simulink model "motorCooling"  (R2022b)
settings: Solver=VariableStepAuto  StartTime=0.0  StopTime=80  RelTol=1e-3  AbsTol=1e-3
PreLoadFcn:
  | load fsDCycle.mat
  | vehicleData
undefined symbols (not defined in the file or in its folder): battery, bevGear, bevMotorSpdRef, cooling, FL, FR, motorDrive, RL, RR, vehicle
libraries: fl_lib x47, nesl_utility x24, sdl_lib x11, SimscapeFluids_lib x3, ee_lib x2, simulink x1, slpidlib x1, autolibshared x1, batteryecm_lib x1, BatteryEstimators x1
(part 3 of 3)

== system motorCooling/Vehicle/Electric Powertrain/SOC ==
  Constant1 : Constant  Value=battery.init_soc
  Current Sensor : fl_lib/Electrical/Electrical Sensors/Current Sensor
  Gain : Gain  Gain=-1
  PS-Simulink Converter1 : nesl_utility/PS-Simulink Converter  PhysicalDomain=network_engine_domain  SubClassName=ps_output  LeftPortType=input  RightPortType=output  PseudoPeriodic=off  Frequencies=[]  VectorFormat=1-D array  Unit=A  AffineConversion=off
  SOC Estimator (Coulomb Counting) : BatteryEstimators/SOC Estimator (Coulomb Counting)  AH=20  Ts=-1
      link override Integrator: LabelModeActiveChoice=Discrete
      settings: LibrarySourceBlock=|
      | batt_sl_lib/Estimators/SOC Estimator
      | (Coulomb Counting)
  + : PMIOPort  Side=Left
  - : PMIOPort  Port=2  Side=Right
  tag scope: SOC=global
  wires:
  Constant1/1 -> SOC Estimator (Coulomb Counting)/2
  SOC Estimator (Coulomb Counting)/1 -> [SOC]  "SOC"
  Gain/1 -> SOC Estimator (Coulomb Counting)/1
  PS-Simulink Converter1/1 -> Gain/1
  connections:
  Current Sensor/RConn2 -- -/RConn1
  PS-Simulink Converter1/LConn1 -- Current Sensor/RConn1
  Current Sensor/LConn1 -- +/RConn1

== system motorCooling/Vehicle/Electric Powertrain/Speed Sensor ==
  Mechanical Rotational Reference1 : fl_lib/Mechanical/Rotational Elements/Mechanical Rotational Reference
  Motion Sensor : fl_lib/Mechanical/Mechanical Sensors/Ideal Rotational Motion Sensor  reference=foundation.enum.MeasurementReference.difference  acceleration_port=false  velocity_port=true  position_port=true  wrap_angle=simscape.enum.onoff.off  offset=0 rad
  PS Terminator : fl_lib/Physical Signals/Sinks/PS Terminator
  PS-Simulink Converter 2 : nesl_utility/PS-Simulink Converter  PhysicalDomain=network_engine_domain  SubClassName=ps_output  LeftPortType=input  RightPortType=output  PseudoPeriodic=off  Frequencies=[]  VectorFormat=1-D array  Unit=rpm  AffineConversion=off
  R : PMIOPort  Side=Left
  w : Outport
  wires:
  PS-Simulink Converter 2/1 -> w/1
  connections:
  Motion Sensor/RConn2 -- PS-Simulink Converter 2/LConn1
  Motion Sensor/RConn1 -- Mechanical Rotational Reference1/LConn1
  Motion Sensor/RConn3 -- PS Terminator/LConn1
  Motion Sensor/LConn1 -- R/RConn1

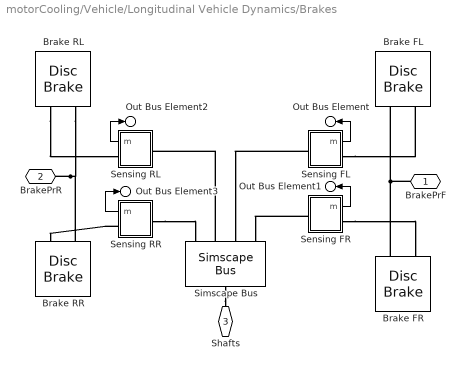
== system motorCooling/Vehicle/Longitudinal Vehicle Dynamics/Brakes ==
  Brake FL : sdl_lib/Brakes & Detents/Rotational/Disc Brake  r_mean=brake.padRadius mm  bore=brake.cylinderBore mm  n_pads=1  thermal_port=simscape.enum.thermaleffects.omit  mu_static=brake.sf  mu_coulomb=brake.cf  temperature_TLU=[280, 300, 320] K  mu_static_TLU=[.9, .8, .7]  mu_coulomb_TLU=[.8, .7, .6]  brkwy_vel=brake.frictionVel rad/s  visc_coef=brake.vfc N*m*s/rad  enable_faults=simscape.enum.onoff.off  faulted_pressure=0 bar  external_fault=simscape.enum.onoff.off  temporal_fault=simscape.enum.onoff.off  fault_time=5 s  report_fault=simscape.enum.assert.action.none  thermal_mass=50 kJ/K  temperature_specify=off  temperature_priority=High  temperature=300 K  temperature_nominal_specify=off  temperature_nominal_unit=K  temperature_nominal_value=1
  Brake FR : sdl_lib/Brakes & Detents/Rotational/Disc Brake  r_mean=brake.padRadius mm  bore=brake.cylinderBore mm  n_pads=1  thermal_port=simscape.enum.thermaleffects.omit  mu_static=brake.sf  mu_coulomb=brake.cf  temperature_TLU=[280, 300, 320] K  mu_static_TLU=[.9, .8, .7]  mu_coulomb_TLU=[.8, .7, .6]  brkwy_vel=brake.frictionVel rad/s  visc_coef=brake.vfc N*m*s/rad  enable_faults=simscape.enum.onoff.off  faulted_pressure=0 bar  external_fault=simscape.enum.onoff.off  temporal_fault=simscape.enum.onoff.off  fault_time=5 s  report_fault=simscape.enum.assert.action.none  thermal_mass=50 kJ/K  temperature_specify=off  temperature_priority=High  temperature=300 K  temperature_nominal_specify=off  temperature_nominal_unit=K  temperature_nominal_value=1
  Brake RL : sdl_lib/Brakes & Detents/Rotational/Disc Brake  r_mean=brake.padRadius mm  bore=brake.cylinderBore mm  n_pads=1  thermal_port=simscape.enum.thermaleffects.omit  mu_static=brake.sf  mu_coulomb=brake.cf  temperature_TLU=[280, 300, 320] K  mu_static_TLU=[.9, .8, .7]  mu_coulomb_TLU=[.8, .7, .6]  brkwy_vel=brake.frictionVel rad/s  visc_coef=brake.vfc N*m*s/rad  enable_faults=simscape.enum.onoff.off  faulted_pressure=0 bar  external_fault=simscape.enum.onoff.off  temporal_fault=simscape.enum.onoff.off  fault_time=5 s  report_fault=simscape.enum.assert.action.none  thermal_mass=50 kJ/K  temperature_specify=off  temperature_priority=High  temperature=300 K  temperature_nominal_specify=off  temperature_nominal_unit=K  temperature_nominal_value=1
  Brake RR : sdl_lib/Brakes & Detents/Rotational/Disc Brake  r_mean=brake.padRadius mm  bore=brake.cylinderBore mm  n_pads=1  thermal_port=simscape.enum.thermaleffects.omit  mu_static=brake.sf  mu_coulomb=brake.cf  temperature_TLU=[280, 300, 320] K  mu_static_TLU=[.9, .8, .7]  mu_coulomb_TLU=[.8, .7, .6]  brkwy_vel=brake.frictionVel rad/s  visc_coef=brake.vfc N*m*s/rad  enable_faults=simscape.enum.onoff.off  faulted_pressure=0 bar  external_fault=simscape.enum.onoff.off  temporal_fault=simscape.enum.onoff.off  fault_time=5 s  report_fault=simscape.enum.assert.action.none  thermal_mass=50 kJ/K  temperature_specify=off  temperature_priority=High  temperature=300 K  temperature_nominal_specify=off  temperature_nominal_unit=K  temperature_nominal_value=1
  Sensing FL : Subsystem
  Sensing FR : Subsystem
  Sensing RL : Subsystem
  Sensing RR : Subsystem
  Simscape Bus : SimscapeBus  HierarchyStrings=RR;RL;FL;FR
  BrakePrF : PMIOPort  Side=Left
  BrakePrR : PMIOPort  Port=2  Side=Left
  Shafts : PMIOPort  Port=3  Side=Right
  Out Bus Element : Outport  PortName=m  Element=FL
  Out Bus Element1 : Outport  PortName=m  Element=FR
  Out Bus Element2 : Outport  PortName=m  Element=RL
  Out Bus Element3 : Outport  PortName=m  Element=RR
  wires:
  Sensing FL/1(m) -> Out Bus Element/1
  Sensing FR/1(m) -> Out Bus Element1/1
  Sensing RL/1(m) -> Out Bus Element2/1
  Sensing RR/1(m) -> Out Bus Element3/1
  connections:
  BrakePrR/RConn1 -- Brake RL/LConn1 -- Brake RR/LConn1
  Brake FR/LConn1 -- Brake FL/LConn1 -- BrakePrF/RConn1
  Sensing FL/LConn1 -- Simscape Bus/LConn3
  Sensing FR/LConn1 -- Simscape Bus/LConn4
  Simscape Bus/LConn2 -- Sensing RL/LConn1
  Sensing RR/LConn1 -- Simscape Bus/LConn1
  Simscape Bus/RConn1 -- Shafts/RConn1
  Sensing FL/RConn1 -- Brake FL/LConn2
  Sensing FR/RConn1 -- Brake FR/LConn2
  Brake RL/LConn2 -- Sensing RL/RConn1
  Sensing RR/RConn1 -- Brake RR/LConn2

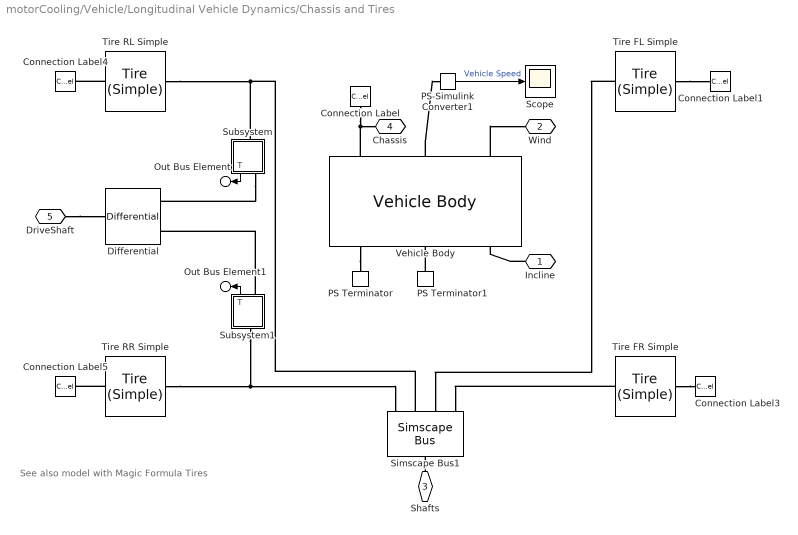
== system motorCooling/Vehicle/Longitudinal Vehicle Dynamics/Chassis and Tires ==
  note: See also model with Magic Formula Tires
  Connection Label{,1,3..5} (5 alike) : ConnectionLabel  Label=VehicleHub
  Differential : sdl_lib/Gears/Differential  driveshaft_location=sdl.enum.differential_orientation.right  cd_ratio=bevGear.gearRatio  friction_model=sdl.enum.gear_friction.none  efficiency=[.85, .92]  temperature_TLU=[280, 300, 320] K  efficiency_ss_TLU=[.95, .9, .85]  efficiency_cd_TLU=[.95, .9, .85]  pwr_thr=[.001, .001] W  mu_visc=[0, 0] N*m*s/rad  model_inertia=simscape.enum.onoff.off  carrier_inertia=0.001 kg*m^2  planet_inertia=0.001 kg*m^2  thermal_mass=50 J/K  T_init=300 K
  PS Terminator : fl_lib/Physical Signals/Sinks/PS Terminator
  PS Terminator1 : fl_lib/Physical Signals/Sinks/PS Terminator
  PS-Simulink Converter1 : nesl_utility/PS-Simulink Converter  PhysicalDomain=network_engine_domain  SubClassName=ps_output  LeftPortType=input  RightPortType=output  PseudoPeriodic=off  Frequencies=[]  VectorFormat=1-D array  Unit=1  AffineConversion=off
  Scope : Scope
  Simscape Bus1 : SimscapeBus  HierarchyStrings=RR;RL;FL;FR
  Subsystem : Subsystem
  Subsystem1 : Subsystem
  Tire FL Simple : sdl_lib/Tires & Vehicles/Tire (Simple)  r_tire=vehicle.tireRollingRadius_cm cm  model_compliance=sdl.enum.compliance.off  stiffness=1e6 N/m  damping=1000 N*s/m  model_inertia=sdl.enum.model_inertia.off  tire_inertia=1 kg*m^2  initial_velocity=0 rad/s
      settings: InternalSimscapePortConfiguration="{\"Bottom\":[],\"Left\":[{\"id\":\"A\",\"label\":\"A\",\"type\":\"foundation.mechanical.rotational.rotational\"}],\"Right\":[{\"id\":\"H\",\"label\":\"H\",\"type\":\"foundation.mechanical.translational.translational\"}],\"Top\":[]}"
  Tire FR Simple : sdl_lib/Tires & Vehicles/Tire (Simple)  r_tire=vehicle.tireRollingRadius_cm cm  model_compliance=sdl.enum.compliance.off  stiffness=1e6 N/m  damping=1000 N*s/m  model_inertia=sdl.enum.model_inertia.off  tire_inertia=1 kg*m^2  initial_velocity=0 rad/s
      settings: InternalSimscapePortConfiguration="{\"Bottom\":[],\"Left\":[{\"id\":\"A\",\"label\":\"A\",\"type\":\"foundation.mechanical.rotational.rotational\"}],\"Right\":[{\"id\":\"H\",\"label\":\"H\",\"type\":\"foundation.mechanical.translational.translational\"}],\"Top\":[]}"
  Tire RL Simple : sdl_lib/Tires & Vehicles/Tire (Simple)  r_tire=vehicle.tireRollingRadius_cm cm  model_compliance=sdl.enum.compliance.off  stiffness=1e6 N/m  damping=1000 N*s/m  model_inertia=sdl.enum.model_inertia.off  tire_inertia=1 kg*m^2  initial_velocity=0 rad/s
      settings: InternalSimscapePortConfiguration="{\"Bottom\":[],\"Left\":[{\"id\":\"A\",\"label\":\"A\",\"type\":\"foundation.mechanical.rotational.rotational\"}],\"Right\":[{\"id\":\"H\",\"label\":\"H\",\"type\":\"foundation.mechanical.translational.translational\"}],\"Top\":[]}"
  Tire RR Simple : sdl_lib/Tires & Vehicles/Tire (Simple)  r_tire=vehicle.tireRollingRadius_cm cm  model_compliance=sdl.enum.compliance.off  stiffness=1e6 N/m  damping=1000 N*s/m  model_inertia=sdl.enum.model_inertia.off  tire_inertia=1 kg*m^2  initial_velocity=0 rad/s
      settings: InternalSimscapePortConfiguration="{\"Bottom\":[],\"Left\":[{\"id\":\"A\",\"label\":\"A\",\"type\":\"foundation.mechanical.rotational.rotational\"}],\"Right\":[{\"id\":\"H\",\"label\":\"H\",\"type\":\"foundation.mechanical.translational.translational\"}],\"Top\":[]}"
  Vehicle Body : sdl_lib/Tires & Vehicles/Vehicle Body  mass=vehicle.riderMass + vehicle.vehicleMass kg  n_w=2  x_f=vehicle.frontAxleDis mm  x_r=vehicle.rearAxleDis mm  y_c=vehicle.cgHeight mm  mass_var=simscape.enum.onoff.off  g=9.81 m/s^2  liftoff_warning=simscape.enum.onoff.off  area=vehicle.frontalArea m^2  Cd=vehicle.cd  rho=1.18 kg/m^3  model_pitch=simscape.enum.onoff.off  inertia=4000 kg*m^2  suspension_model=sdl.enum.linearTLU.linear  k_f=1e4 N/m  b_f=1e4 N*s/m  k_r=1e4 N/m  b_r=1e4 N*s/m  k_f_TLU=[-2000, -1000, 0, 1000, 2000] N  x_f_TLU=[-.4, -.2, 0, .2, .4] m  b_f_TLU=[-200, -100, 0, 100, 200] N  v_f_TLU=[-4, -2, 0, 2, 4] m/s  k_r_TLU=[-2000, -1000, 0, 1000, 2000] N  x_r_TLU=[-.4, -.2, 0, .2, .4] m  b_r_TLU=[-200, -100, 0, 100, 200] N  v_r_TLU=[-4, -2, 0, 2, 4] m/s  interp_method=simscape.enum.interpolation.linear  extrap_method=simscape.enum.extrapolation.linear  model_hardstop=simscape.enum.onoff.off  upper_bound_f=.25 m  lower_bound_f=-.25 m  stop_k_f=1e6 N/m  stop_b_f=150 N*s/m  upper_bound_r=.25 m  lower_bound_r=-.25 m  stop_k_r=1e6 N/m  stop_b_r=150 N*s/m  initial_pitch=0 rad  initial_pitch_rate=0 rad/s  v_specify=off  v_priority=High  v=12.95 m/s  v_nominal_specify=off  v_nominal_unit=m/s  v_nominal_value=1
  Incline : PMIOPort  Side=Right
  Wind : PMIOPort  Port=2  Side=Right
  Shafts : PMIOPort  Port=3  Side=Left
  Chassis : PMIOPort  Port=4  Side=Right
  DriveShaft : PMIOPort  Port=5  Side=Left
  Out Bus Element : Outport  PortName=m  Element=tRL
  Out Bus Element1 : Outport  PortName=m  Element=tRR
  wires:
  PS-Simulink Converter1/1 -> Scope/1  "Vehicle Speed"
  Subsystem/1(T) -> Out Bus Element/1
  Subsystem1/1(T) -> Out Bus Element1/1
  connections:
  Tire RR Simple/RConn1 -- Connection Label5/LConn1
  Tire FL Simple/RConn1 -- Connection Label1/LConn1
  Tire RL Simple/RConn1 -- Connection Label4/LConn1
  Vehicle Body/LConn2 -- PS-Simulink Converter1/LConn1
  Tire FR Simple/RConn1 -- Connection Label3/LConn1
  Tire FR Simple/LConn1 -- Simscape Bus1/LConn4
  DriveShaft/RConn1 -- Differential/LConn1
  Connection Label/LConn1 -- Vehicle Body/LConn1 -- Chassis/RConn1
  Subsystem1/LConn1 -- Tire RR Simple/LConn1 -- Simscape Bus1/LConn1
  Tire FL Simple/LConn1 -- Simscape Bus1/LConn3
  Simscape Bus1/LConn2 -- Tire RL Simple/LConn1 -- Subsystem/LConn1
  Shafts/RConn1 -- Simscape Bus1/RConn1
  Incline/RConn1 -- Vehicle Body/RConn3
  Vehicle Body/LConn3 -- Wind/RConn1
  Subsystem1/RConn1 -- Differential/RConn1
  Subsystem/RConn1 -- Differential/RConn2
  Vehicle Body/RConn1 -- PS Terminator/LConn1
  PS Terminator1/LConn1 -- Vehicle Body/RConn2

== system motorCooling/Vehicle/Longitudinal Vehicle Dynamics/Env ==
  m : Inport
  Road Grade (rad) : Constant  Value=0
  Signal Specification : SignalSpecification  Unit=rad
  Terminator : Terminator
  Wind (m/s) : Constant  Value=0
  Bus Element Out2 : Outport  PortName=Env  Element=RoadGrade
      settings: AttributesFormatString=%<Unit>
  Bus Element Out4 : Outport  PortName=Env  Element=Wind
      settings: AttributesFormatString=%<Unit>
  wires:
  Wind (m/s)/1 -> Bus Element Out4/1
  m/1 -> Terminator/1
  Road Grade (rad)/1 -> Signal Specification/1
  Signal Specification/1 -> Bus Element Out2/1

== system motorCooling/Vehicle/Longitudinal Vehicle Dynamics/Pressure Drag ==
  Vel : Inport
  Gain : Gain  Gain=0.5*cooling.cDrag*cooling.denAir
  Simulink-PS Converter : nesl_utility/Simulink-PS Converter  PhysicalDomain=network_engine_domain  SubClassName=ps_input  LeftPortType=input  RightPortType=output  PseudoPeriodic=off  Frequencies=[]  NoiseDistribution=none  NoiseParameters=[]  Unit=Pa  AffineConversion=off  FilteringAndDerivatives=provide  SimscapeFilterOrder=1  InputFilterTimeConstant=0.001  UdotUserProvided=0
  Square : Math  Operator=square
  Transfer Fcn : TransferFcn  Denominator=[0.5 1]
  Pressure : PMIOPort  Side=Right
  wires:
  Vel/1 -> Square/1
  Gain/1 -> Transfer Fcn/1
  Square/1 -> Gain/1
  Transfer Fcn/1 -> Simulink-PS Converter/1
  connections:
  Simulink-PS Converter/RConn1 -- Pressure/RConn1

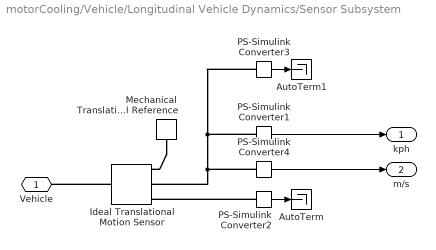
== system motorCooling/Vehicle/Longitudinal Vehicle Dynamics/Sensor Subsystem ==
  AutoTerm : Terminator
  AutoTerm1 : Terminator
  Ideal Translational Motion Sensor : fl_lib/Mechanical/Mechanical Sensors/Ideal Translational Motion Sensor  reference=foundation.enum.MeasurementReference.difference  acceleration_port=false  velocity_port=true  position_port=true  offset=0 m
  Mechanical Translational Reference : fl_lib/Mechanical/Translational Elements/Mechanical Translational Reference
  PS-Simulink Converter1 : nesl_utility/PS-Simulink Converter  PhysicalDomain=network_engine_domain  SubClassName=ps_output  LeftPortType=input  RightPortType=output  PseudoPeriodic=off  Frequencies=[]  VectorFormat=1-D array  Unit=km/hr  AffineConversion=off
  PS-Simulink Converter2 : nesl_utility/PS-Simulink Converter  PhysicalDomain=network_engine_domain  SubClassName=ps_output  LeftPortType=input  RightPortType=output  PseudoPeriodic=off  Frequencies=[]  VectorFormat=1-D array  Unit=1  AffineConversion=off
  PS-Simulink Converter3 : nesl_utility/PS-Simulink Converter  PhysicalDomain=network_engine_domain  SubClassName=ps_output  LeftPortType=input  RightPortType=output  PseudoPeriodic=off  Frequencies=[]  VectorFormat=1-D array  Unit=mph  AffineConversion=off
  PS-Simulink Converter4 : nesl_utility/PS-Simulink Converter  PhysicalDomain=network_engine_domain  SubClassName=ps_output  LeftPortType=input  RightPortType=output  PseudoPeriodic=off  Frequencies=[]  VectorFormat=1-D array  Unit=m/s  AffineConversion=off
  Vehicle : PMIOPort  Side=Left
  kph : Outport  VectorParamsAs1DForOutWhenUnconnected=off
  m/s : Outport  Port=2  VectorParamsAs1DForOutWhenUnconnected=off
  wires:
  PS-Simulink Converter1/1 -> kph/1
  PS-Simulink Converter2/1 -> AutoTerm/1
  PS-Simulink Converter3/1 -> AutoTerm1/1
  PS-Simulink Converter4/1 -> m/s/1
  connections:
  Mechanical Translational Reference/LConn1 -- Ideal Translational Motion Sensor/RConn1
  PS-Simulink Converter2/LConn1 -- Ideal Translational Motion Sensor/RConn3
  Ideal Translational Motion Sensor/LConn1 -- Vehicle/RConn1
  PS-Simulink Converter3/LConn1 -- PS-Simulink Converter4/LConn1 -- Ideal Translational Motion Sensor/RConn2 -- PS-Simulink Converter1/LConn1

== system motorCooling/Vehicle/Electric Powertrain/Motor Cooling System/Sensing Temperature ==
  PS-Simulink Converter : nesl_utility/PS-Simulink Converter  PhysicalDomain=network_engine_domain  SubClassName=ps_output  LeftPortType=input  RightPortType=output  PseudoPeriodic=off  Frequencies=[]  VectorFormat=inherit  Unit=degC  AffineConversion=on
  Temperature Sensor : fl_lib/Thermal/Thermal Sensors/Temperature Sensor
  Thermal Reference : fl_lib/Thermal/Thermal Elements/Thermal Reference
  H : PMIOPort  Side=Left
  T : Outport
  wires:
  PS-Simulink Converter/1 -> T/1  "Motor Temperature"
  connections:
  PS-Simulink Converter/LConn1 -- Temperature Sensor/RConn2
  Thermal Reference/LConn1 -- Temperature Sensor/RConn1
  Temperature Sensor/LConn1 -- H/RConn1

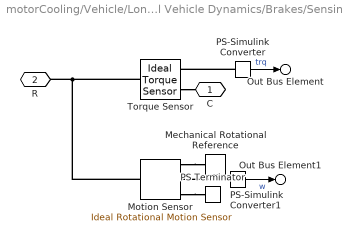
== system motorCooling/Vehicle/Longitudinal Vehicle Dynamics/Brakes/Sensing FL ==
  Mechanical Rotational Reference : fl_lib/Mechanical/Rotational Elements/Mechanical Rotational Reference
  Motion Sensor : fl_lib/Mechanical/Mechanical Sensors/Ideal Rotational Motion Sensor  reference=foundation.enum.MeasurementReference.difference  acceleration_port=false  velocity_port=true  position_port=true  wrap_angle=simscape.enum.onoff.off  offset=0 rad
  PS Terminator : fl_lib/Physical Signals/Sinks/PS Terminator
  PS-Simulink Converter : nesl_utility/PS-Simulink Converter  PhysicalDomain=network_engine_domain  SubClassName=ps_output  LeftPortType=input  RightPortType=output  PseudoPeriodic=off  Frequencies=[]  VectorFormat=inherit  Unit=inherit  AffineConversion=off
  PS-Simulink Converter1 : nesl_utility/PS-Simulink Converter  PhysicalDomain=network_engine_domain  SubClassName=ps_output  LeftPortType=input  RightPortType=output  PseudoPeriodic=off  Frequencies=[]  VectorFormat=inherit  Unit=inherit  AffineConversion=off
  Torque Sensor : fl_lib/Mechanical/Mechanical Sensors/Ideal Torque Sensor
  C : PMIOPort  Side=Left
  R : PMIOPort  Port=2  Side=Right
  Out Bus Element : Outport  PortName=m  Element=brkTrqFL
  Out Bus Element1 : Outport  PortName=m  Element=wFL
  wires:
  PS-Simulink Converter1/1 -> Out Bus Element1/1  "w"
  PS-Simulink Converter/1 -> Out Bus Element/1  "trq"
  connections:
  Motion Sensor/RConn3 -- PS Terminator/LConn1
  PS-Simulink Converter1/LConn1 -- Motion Sensor/RConn2
  Motion Sensor/RConn1 -- Mechanical Rotational Reference/LConn1
  Torque Sensor/RConn1 -- C/RConn1
  Motion Sensor/LConn1 -- Torque Sensor/LConn1 -- R/RConn1
  PS-Simulink Converter/LConn1 -- Torque Sensor/RConn2

== system motorCooling/Vehicle/Longitudinal Vehicle Dynamics/Brakes/Sensing FR ==
  Mechanical Rotational Reference : fl_lib/Mechanical/Rotational Elements/Mechanical Rotational Reference
  Motion Sensor : fl_lib/Mechanical/Mechanical Sensors/Ideal Rotational Motion Sensor  reference=foundation.enum.MeasurementReference.difference  acceleration_port=false  velocity_port=true  position_port=true  wrap_angle=simscape.enum.onoff.off  offset=0 rad
  PS Terminator : fl_lib/Physical Signals/Sinks/PS Terminator
  PS-Simulink Converter : nesl_utility/PS-Simulink Converter  PhysicalDomain=network_engine_domain  SubClassName=ps_output  LeftPortType=input  RightPortType=output  PseudoPeriodic=off  Frequencies=[]  VectorFormat=inherit  Unit=inherit  AffineConversion=off
  PS-Simulink Converter1 : nesl_utility/PS-Simulink Converter  PhysicalDomain=network_engine_domain  SubClassName=ps_output  LeftPortType=input  RightPortType=output  PseudoPeriodic=off  Frequencies=[]  VectorFormat=inherit  Unit=inherit  AffineConversion=off
  Torque Sensor : fl_lib/Mechanical/Mechanical Sensors/Ideal Torque Sensor
  C : PMIOPort  Side=Left
  R : PMIOPort  Port=2  Side=Right
  Out Bus Element : Outport  PortName=m  Element=brkTrqFR
  Out Bus Element1 : Outport  PortName=m  Element=wFR
  wires:
  PS-Simulink Converter/1 -> Out Bus Element/1  "trq"
  PS-Simulink Converter1/1 -> Out Bus Element1/1  "w"
  connections:
  PS-Simulink Converter/LConn1 -- Torque Sensor/RConn2
  R/RConn1 -- Torque Sensor/LConn1 -- Motion Sensor/LConn1
  Torque Sensor/RConn1 -- C/RConn1
  Motion Sensor/RConn1 -- Mechanical Rotational Reference/LConn1
  PS-Simulink Converter1/LConn1 -- Motion Sensor/RConn2
  Motion Sensor/RConn3 -- PS Terminator/LConn1

== system motorCooling/Vehicle/Longitudinal Vehicle Dynamics/Brakes/Sensing RL ==
  Mechanical Rotational Reference : fl_lib/Mechanical/Rotational Elements/Mechanical Rotational Reference
  Motion Sensor : fl_lib/Mechanical/Mechanical Sensors/Ideal Rotational Motion Sensor  reference=foundation.enum.MeasurementReference.difference  acceleration_port=false  velocity_port=true  position_port=true  wrap_angle=simscape.enum.onoff.off  offset=0 rad
  PS Terminator : fl_lib/Physical Signals/Sinks/PS Terminator
  PS-Simulink Converter : nesl_utility/PS-Simulink Converter  PhysicalDomain=network_engine_domain  SubClassName=ps_output  LeftPortType=input  RightPortType=output  PseudoPeriodic=off  Frequencies=[]  VectorFormat=inherit  Unit=inherit  AffineConversion=off
  PS-Simulink Converter1 : nesl_utility/PS-Simulink Converter  PhysicalDomain=network_engine_domain  SubClassName=ps_output  LeftPortType=input  RightPortType=output  PseudoPeriodic=off  Frequencies=[]  VectorFormat=inherit  Unit=inherit  AffineConversion=off
  Torque Sensor : fl_lib/Mechanical/Mechanical Sensors/Ideal Torque Sensor
  C : PMIOPort  Side=Left
  R : PMIOPort  Port=2  Side=Right
  Out Bus Element : Outport  PortName=m  Element=brkTrqRL
  Out Bus Element1 : Outport  PortName=m  Element=wRL
  wires:
  PS-Simulink Converter/1 -> Out Bus Element/1  "trq"
  PS-Simulink Converter1/1 -> Out Bus Element1/1  "w"
  connections:
  PS-Simulink Converter/LConn1 -- Torque Sensor/RConn2
  Torque Sensor/LConn1 -- Motion Sensor/LConn1 -- R/RConn1
  Torque Sensor/RConn1 -- C/RConn1
  Motion Sensor/RConn1 -- Mechanical Rotational Reference/LConn1
  PS-Simulink Converter1/LConn1 -- Motion Sensor/RConn2
  Motion Sensor/RConn3 -- PS Terminator/LConn1

== system motorCooling/Vehicle/Longitudinal Vehicle Dynamics/Brakes/Sensing RR ==
  Mechanical Rotational Reference : fl_lib/Mechanical/Rotational Elements/Mechanical Rotational Reference
  Motion Sensor : fl_lib/Mechanical/Mechanical Sensors/Ideal Rotational Motion Sensor  reference=foundation.enum.MeasurementReference.difference  acceleration_port=false  velocity_port=true  position_port=true  wrap_angle=simscape.enum.onoff.off  offset=0 rad
  PS Terminator : fl_lib/Physical Signals/Sinks/PS Terminator
  PS-Simulink Converter : nesl_utility/PS-Simulink Converter  PhysicalDomain=network_engine_domain  SubClassName=ps_output  LeftPortType=input  RightPortType=output  PseudoPeriodic=off  Frequencies=[]  VectorFormat=inherit  Unit=inherit  AffineConversion=off
  PS-Simulink Converter1 : nesl_utility/PS-Simulink Converter  PhysicalDomain=network_engine_domain  SubClassName=ps_output  LeftPortType=input  RightPortType=output  PseudoPeriodic=off  Frequencies=[]  VectorFormat=inherit  Unit=inherit  AffineConversion=off
  Torque Sensor : fl_lib/Mechanical/Mechanical Sensors/Ideal Torque Sensor
  C : PMIOPort  Side=Left
  R : PMIOPort  Port=2  Side=Right
  Out Bus Element : Outport  PortName=m  Element=brqTrqRR
  Out Bus Element1 : Outport  PortName=m  Element=wRR
  wires:
  PS-Simulink Converter1/1 -> Out Bus Element1/1  "w"
  PS-Simulink Converter/1 -> Out Bus Element/1  "trq"
  connections:
  Motion Sensor/RConn3 -- PS Terminator/LConn1
  PS-Simulink Converter1/LConn1 -- Motion Sensor/RConn2
  Motion Sensor/RConn1 -- Mechanical Rotational Reference/LConn1
  Torque Sensor/RConn1 -- C/RConn1
  Motion Sensor/LConn1 -- Torque Sensor/LConn1 -- R/RConn1
  PS-Simulink Converter/LConn1 -- Torque Sensor/RConn2

== system motorCooling/Vehicle/Longitudinal Vehicle Dynamics/Chassis and Tires/Subsystem ==
  PS-Simulink Converter : nesl_utility/PS-Simulink Converter  PhysicalDomain=network_engine_domain  SubClassName=ps_output  LeftPortType=input  RightPortType=output  PseudoPeriodic=off  Frequencies=[]  VectorFormat=inherit  Unit=inherit  AffineConversion=off
  Torque Sensor Motor RL : fl_lib/Mechanical/Mechanical Sensors/Ideal Torque Sensor
  C : PMIOPort  Side=Left
  R : PMIOPort  Port=2  Side=Right
  T : Outport
  wires:
  PS-Simulink Converter/1 -> T/1
  connections:
  Torque Sensor Motor RL/RConn1 -- C/RConn1
  Torque Sensor Motor RL/LConn1 -- R/RConn1
  PS-Simulink Converter/LConn1 -- Torque Sensor Motor RL/RConn2

== system motorCooling/Vehicle/Longitudinal Vehicle Dynamics/Chassis and Tires/Subsystem1 ==
  PS-Simulink Converter : nesl_utility/PS-Simulink Converter  PhysicalDomain=network_engine_domain  SubClassName=ps_output  LeftPortType=input  RightPortType=output  PseudoPeriodic=off  Frequencies=[]  VectorFormat=inherit  Unit=inherit  AffineConversion=off
  Torque Sensor Motor RL : fl_lib/Mechanical/Mechanical Sensors/Ideal Torque Sensor
  C : PMIOPort  Side=Left
  R : PMIOPort  Port=2  Side=Right
  T : Outport
  wires:
  PS-Simulink Converter/1 -> T/1
  connections:
  PS-Simulink Converter/LConn1 -- Torque Sensor Motor RL/RConn2
  Torque Sensor Motor RL/LConn1 -- R/RConn1
  Torque Sensor Motor RL/RConn1 -- C/RConn1
